simulink model "mod_bio"  (R2017a)
settings: Solver=ode45  StartTime=0.0  StopTime=100  RelTol=1e-3  EnableMultiTasking=on
settings Model: Creator=Tanay  LastModifiedBy=pum
settings DataIOCC: LimitDataPoints=on  SaveFormat=Array
settings OptimizationCC: LifeSpan=inf
settings DebuggingCC: SolverPrmCheckMsg=warning  SFUnexpectedBacktrackingDiag=warning  SFNoUnconditionalDefaultTransitionDiag=warning  SFExecutionAtInitializationDiag=none
settings HardwareCC: ProdBitPerPointer=32  ProdBitPerSizeT=32  ProdBitPerPtrDiffT=32  ProdLargestAtomicFloat=None  ProdIntDivRoundTo=Undefined  ProdEndianess=Unspecified  ProdWordSize=32  ProdHWDeviceType=32-bit Generic
settings ModelReferenceCC: PropagateSignalLabelsOutOfModel=off
settings GRTTargetCC: TargetLangStandard=C89/C90 (ANSI)  GeneratePreprocessorConditionals=Disable all
settings ConfigComp: CovMetricSettings=dw  CovHtmlReporting=on  CovSaveCumulativeToWorkspaceVar=on  CovSaveSingleToWorkspaceVar=on  CovExternalEMLEnable=off  CovSFcnEnable=off

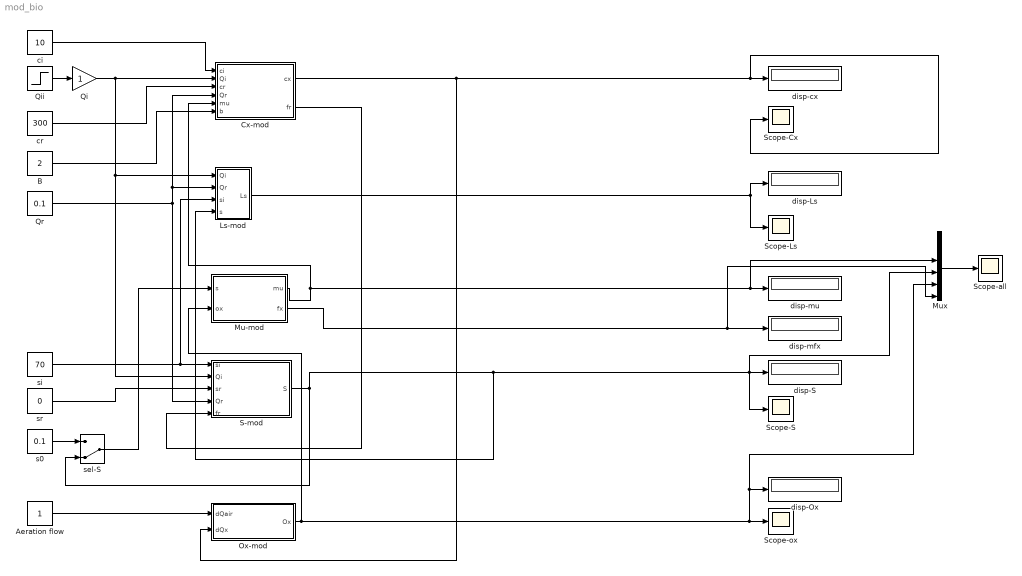
== system mod_bio ==
  Aeration flow : Constant
  B : Constant  Value=2
  Cx-mod : Subsystem  mask{V=5}
      mask prompts: V "Volume"
  Ls-mod : Subsystem  mask{V=5, Z=0.25}
      mask prompts: V "Volume"
  Mu-mod : Subsystem  mask{mu_max=6, K=5, wf=1, wo=2, sx_lim=36, sx_max=40}
      mask prompts: mu_max "Maximum"; K "Dropness"; wf "Feed weight"; wo "Oxygen weight"; sx_lim "Overfeed"; sx_max "Deadfeed"
  Mux : Mux  Inputs=6
  Ox-mod : Subsystem  mask{ox_max=10, ox_min=2, alpha=0.5, beta=2, gamma=0.01}
      mask prompts: ox_max "Maximum"; ox_min "Minimum"; alpha "Coef. aeration"; beta "Coef. de-aeration"; gamma "Coef. consumption"
  Qi : Gain
  Qii : Step  SampleTime=0
  Qr : Constant  Value=0.1
  S-mod : Subsystem  mask{V=5, Y=0.01}
      mask prompts: V "Volume"; Y "Regeneration"
  Scope-Cx : Scope
  Scope-Ls : Scope
  Scope-S : Scope
  Scope-all : Scope
  Scope-ox : Scope
  ci : Constant  Value=10
  cr : Constant  Value=300
  disp-Ls : Display
  disp-Ox : Display
  disp-S : Display
  disp-cx : Display
  disp-mfx : Display
  disp-mu : Display
  s0 : Constant  Value=0.1
  sel-S : ManualSwitch  CurrentSetting=0
  si : Constant  Value=70
  sr : Constant  Value=0
  wires:
  ci/1 -> Cx-mod/1(ci)
  Qii/1 -> Qi/1
  cr/1 -> Cx-mod/3(cr)
  Qr/1 -> Cx-mod/4(Qr), Ls-mod/2(Qr), S-mod/4(Qr)
  B/1 -> Cx-mod/6(b)
  Cx-mod/1(cx) -> Ox-mod/2(dQx), Scope-Cx/1, disp-cx/1
  s0/1 -> sel-S/1
  si/1 -> S-mod/1(si), Ls-mod/3(si)
  sr/1 -> S-mod/3(sr)
  Cx-mod/2(fr) -> S-mod/5(fr)
  sel-S/1 -> Mu-mod/1(s)
  Qi/1 -> Ls-mod/1(Qi), S-mod/2(Qi), Cx-mod/2(Qi)
  Ls-mod/1(Ls) -> disp-Ls/1, Scope-Ls/1
  Aeration flow/1 -> Ox-mod/1(dQair)
  Ox-mod/1(Ox) -> disp-Ox/1, Mux/5, Scope-ox/1, Mu-mod/2(ox)
  Mu-mod/2(fx) -> Mux/6, disp-mfx/1
  S-mod/1(S) -> Ls-mod/4(s), Mux/4, Scope-S/1, disp-S/1, sel-S/2
  Mu-mod/1(mu) -> Cx-mod/5(mu), Mux/3, disp-mu/1
  Mux/1 -> Scope-all/1

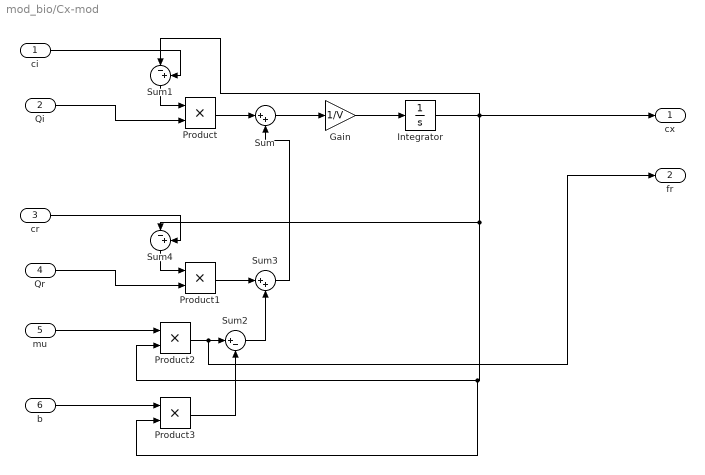
== system mod_bio/Cx-mod ==
  ci : Inport
  Qi : Inport  Port=2
  cr : Inport  Port=3
  Qr : Inport  Port=4
  mu : Inport  Port=5
  b : Inport  Port=6
  Gain : Gain  Gain=1/V
  Integrator : Integrator
  Product{,1..3} (4 alike) : Product
  Sum : Sum  Inputs=|++
  Sum1 : Sum  Inputs=|-+
  Sum2 : Sum  Inputs=|+-
  Sum3 : Sum  Inputs=|++
  Sum4 : Sum  Inputs=|-+
  cx : Outport
  fr : Outport  Port=2
  wires:
  Sum4/1 -> Product1/1
  Product3/1 -> Sum2/2
  Sum2/1 -> Sum3/2
  Integrator/1 -> cx/1, Product3/2, Product2/2, Sum4/1, Sum1/1
  Product1/1 -> Sum3/1
  Qr/1 -> Product1/2
  cr/1 -> Sum4/2
  Product2/1 -> fr/1, Sum2/1
  b/1 -> Product3/1
  Gain/1 -> Integrator/1
  Sum1/1 -> Product/1
  ci/1 -> Sum1/2
  Sum/1 -> Gain/1
  Qi/1 -> Product/2
  Product/1 -> Sum/1
  mu/1 -> Product2/1
  Sum3/1 -> Sum/2

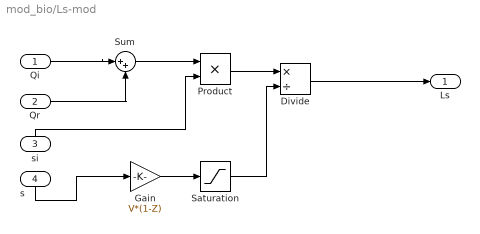
== system mod_bio/Ls-mod ==
  Qi : Inport
  Qr : Inport  Port=2
  si : Inport  Port=3
  s : Inport  Port=4
  Divide : Product  Inputs=*/
  Gain : Gain  Gain=V*(1-Z)
  Product : Product
  Saturation : Saturate  UpperLimit=1e6  LowerLimit=1e-2
  Sum : Sum  Inputs=|++
  Ls : Outport
  wires:
  Gain/1 -> Saturation/1
  Sum/1 -> Product/1
  Product/1 -> Divide/1
  Qr/1 -> Sum/2
  si/1 -> Product/2
  Divide/1 -> Ls/1
  s/1 -> Gain/1
  Qi/1 -> Sum/1
  Saturation/1 -> Divide/2

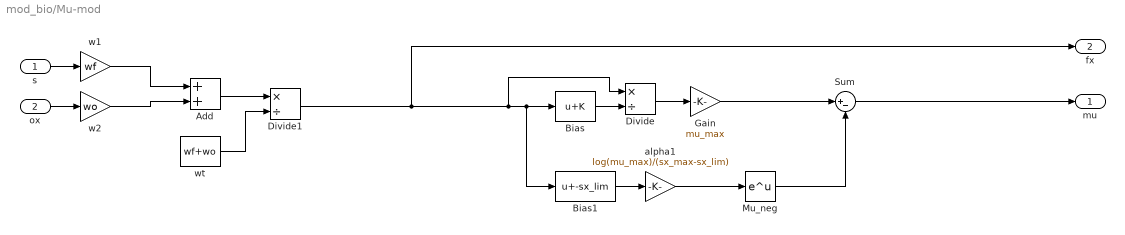
== system mod_bio/Mu-mod ==
  s : Inport
  ox : Inport  Port=2
  Add : Sum
  Bias : Bias  Bias=K
  Bias1 : Bias  Bias=-sx_lim
  Divide : Product  Inputs=*/
  Divide1 : Product  Inputs=*/
  Gain : Gain  Gain=mu_max
  Mu_neg : Math  SaturateOnIntegerOverflow=on
  Sum : Sum  Inputs=|+-
  alpha1 : Gain  Gain=log(mu_max)/(sx_max-sx_lim)
  w1 : Gain  Gain=wf
  w2 : Gain  Gain=wo
  wt : Constant  Value=wf+wo
  mu : Outport
  fx : Outport  Port=2
  wires:
  Gain/1 -> Sum/1
  Bias/1 -> Divide/2
  Divide/1 -> Gain/1
  s/1 -> w1/1
  ox/1 -> w2/1
  w1/1 -> Add/1
  w2/1 -> Add/2
  Add/1 -> Divide1/1
  Divide1/1 -> fx/1, Divide/1, Bias1/1, Bias/1
  wt/1 -> Divide1/2
  Sum/1 -> mu/1
  Mu_neg/1 -> Sum/2
  alpha1/1 -> Mu_neg/1
  Bias1/1 -> alpha1/1

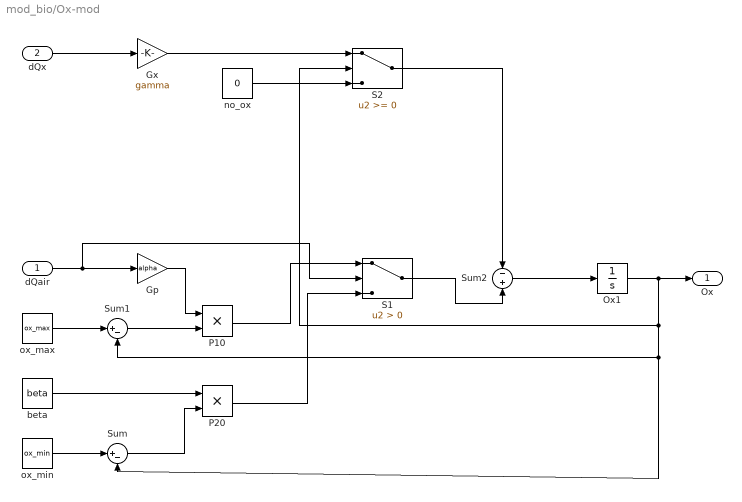
== system mod_bio/Ox-mod ==
  dQair : Inport
  dQx : Inport  Port=2
  Gp : Gain  Gain=alpha
  Gx : Gain  Gain=gamma
  Ox1 : Integrator
  P10 : Product
  P20 : Product
  S1 : Switch  Criteria=u2 > Threshold  ZeroCross=off
  S2 : Switch  ZeroCross=off
  Sum : Sum  Inputs=|+-
  Sum1 : Sum  Inputs=|+-
  Sum2 : Sum  Inputs=-+
  beta : Constant  Value=beta
  no_ox : Constant  Value=0
  ox_max : Constant  Value=ox_max
  ox_min : Constant  Value=ox_min
  Ox : Outport
  wires:
  Ox1/1 -> S2/2, Sum1/2, Sum/2, Ox/1
  ox_max/1 -> Sum1/1
  ox_min/1 -> Sum/1
  S1/1 -> Sum2/2
  dQair/1 -> Gp/1, S1/2
  Sum1/1 -> P10/2
  P10/1 -> S1/1
  Gp/1 -> P10/1
  Sum/1 -> P20/2
  beta/1 -> P20/1
  P20/1 -> S1/3
  Sum2/1 -> Ox1/1
  Gx/1 -> S2/1
  dQx/1 -> Gx/1
  S2/1 -> Sum2/1
  no_ox/1 -> S2/3

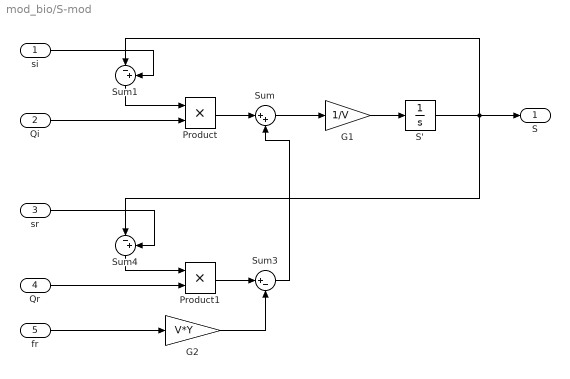
== system mod_bio/S-mod ==
  si : Inport
  Qi : Inport  Port=2
  sr : Inport  Port=3
  Qr : Inport  Port=4
  fr : Inport  Port=5
  G1 : Gain  Gain=1/V
  G2 : Gain  Gain=V*Y
  Product : Product
  Product1 : Product
  S' : Integrator
  Sum : Sum  Inputs=|++
  Sum1 : Sum  Inputs=|-+
  Sum3 : Sum  Inputs=|+-
  Sum4 : Sum  Inputs=|-+
  S : Outport
  wires:
  Sum4/1 -> Product1/1
  G2/1 -> Sum3/2
  S'/1 -> S/1, Sum4/1, Sum1/1
  Product1/1 -> Sum3/1
  Qr/1 -> Product1/2
  sr/1 -> Sum4/2
  G1/1 -> S'/1
  Sum1/1 -> Product/1
  si/1 -> Sum1/2
  Sum/1 -> G1/1
  Qi/1 -> Product/2
  Product/1 -> Sum/1
  fr/1 -> G2/1
  Sum3/1 -> Sum/2
